simulink model "Eng"  (R2018a)
settings: configuration reference "cs_ert" (kept outside this file)
settings Model: DataDictionary=Eng.sldd  Creator=zhoutinglin  LastModifiedBy=zhoutinglin

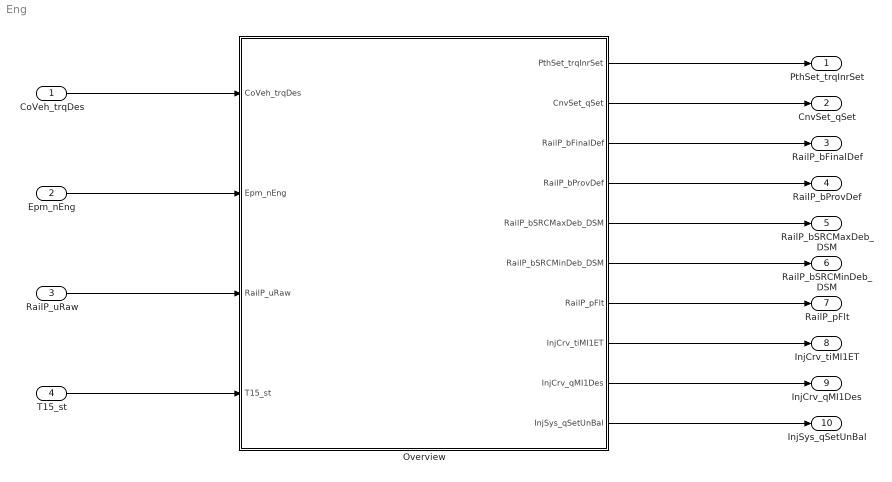
== system Eng ==
  CoVeh_trqDes : Inport
  Epm_nEng : Inport  Port=2
  RailP_uRaw : Inport  Port=3
  T15_st : Inport  Port=4
  Overview : Subsystem
  PthSet_trqInrSet : Outport
  CnvSet_qSet : Outport  Port=2
  RailP_bFinalDef : Outport  Port=3
  RailP_bProvDef : Outport  Port=4
  RailP_bSRCMaxDeb_DSM : Outport  Port=5
  RailP_bSRCMinDeb_DSM : Outport  Port=6
  RailP_pFlt : Outport  Port=7
  InjCrv_tiMI1ET : Outport  Port=8
  InjCrv_qMI1Des : Outport  Port=9
  InjSys_qSetUnBal : Outport  Port=10
  wires:
  CoVeh_trqDes/1 -> Overview/1(CoVeh_trqDes)
  Epm_nEng/1 -> Overview/2(Epm_nEng)
  RailP_uRaw/1 -> Overview/3(RailP_uRaw)
  T15_st/1 -> Overview/4(T15_st)
  Overview/1(PthSet_trqInrSet) -> PthSet_trqInrSet/1
  Overview/2(CnvSet_qSet) -> CnvSet_qSet/1
  Overview/3(RailP_bFinalDef) -> RailP_bFinalDef/1
  Overview/4(RailP_bProvDef) -> RailP_bProvDef/1
  Overview/5(RailP_bSRCMaxDeb_DSM) -> RailP_bSRCMaxDeb_DSM/1
  Overview/6(RailP_bSRCMinDeb_DSM) -> RailP_bSRCMinDeb_DSM/1
  Overview/7(RailP_pFlt) -> RailP_pFlt/1
  Overview/8(InjCrv_tiMI1ET) -> InjCrv_tiMI1ET/1
  Overview/9(InjCrv_qMI1Des) -> InjCrv_qMI1Des/1
  Overview/10(InjSys_qSetUnBal) -> InjSys_qSetUnBal/1

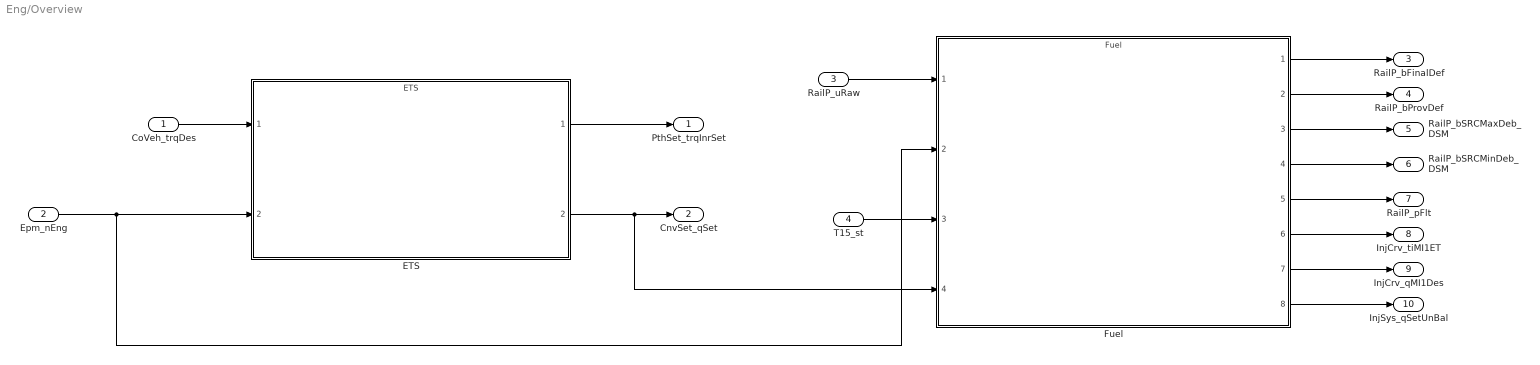
== system Eng/Overview ==
  CoVeh_trqDes : Inport
  Epm_nEng : Inport  Port=2
  RailP_uRaw : Inport  Port=3
  T15_st : Inport  Port=4
  ETS : ModelReference  ModelNameDialog=ETS  SimulationMode=Normal  ModelReferenceVersion=1.2
  Fuel : ModelReference  ModelNameDialog=Fuel  SimulationMode=Normal  ModelReferenceVersion=1.3
  PthSet_trqInrSet : Outport
  CnvSet_qSet : Outport  Port=2
  RailP_bFinalDef : Outport  Port=3
  RailP_bProvDef : Outport  Port=4
  RailP_bSRCMaxDeb_DSM : Outport  Port=5
  RailP_bSRCMinDeb_DSM : Outport  Port=6
  RailP_pFlt : Outport  Port=7
  InjCrv_tiMI1ET : Outport  Port=8
  InjCrv_qMI1Des : Outport  Port=9
  InjSys_qSetUnBal : Outport  Port=10
  wires:
  CoVeh_trqDes/1 -> ETS/1
  Epm_nEng/1 -> Fuel/2, ETS/2
  ETS/1 -> PthSet_trqInrSet/1
  ETS/2 -> Fuel/4, CnvSet_qSet/1
  RailP_uRaw/1 -> Fuel/1
  T15_st/1 -> Fuel/3
  Fuel/1 -> RailP_bFinalDef/1
  Fuel/2 -> RailP_bProvDef/1
  Fuel/3 -> RailP_bSRCMaxDeb_DSM/1
  Fuel/4 -> RailP_bSRCMinDeb_DSM/1
  Fuel/5 -> RailP_pFlt/1
  Fuel/6 -> InjCrv_tiMI1ET/1
  Fuel/7 -> InjCrv_qMI1Des/1
  Fuel/8 -> InjSys_qSetUnBal/1
